simulink model "Nonlinear_model_with_observer"  (Simulink 7.7)
settings: Solver=ode45  StartTime=0.0  StopTime=6  RelTol=1e-3
undefined symbols (not defined in the file or in its folder): quad
settings Model: Creator=Alexey  LastModifiedBy=Alexey

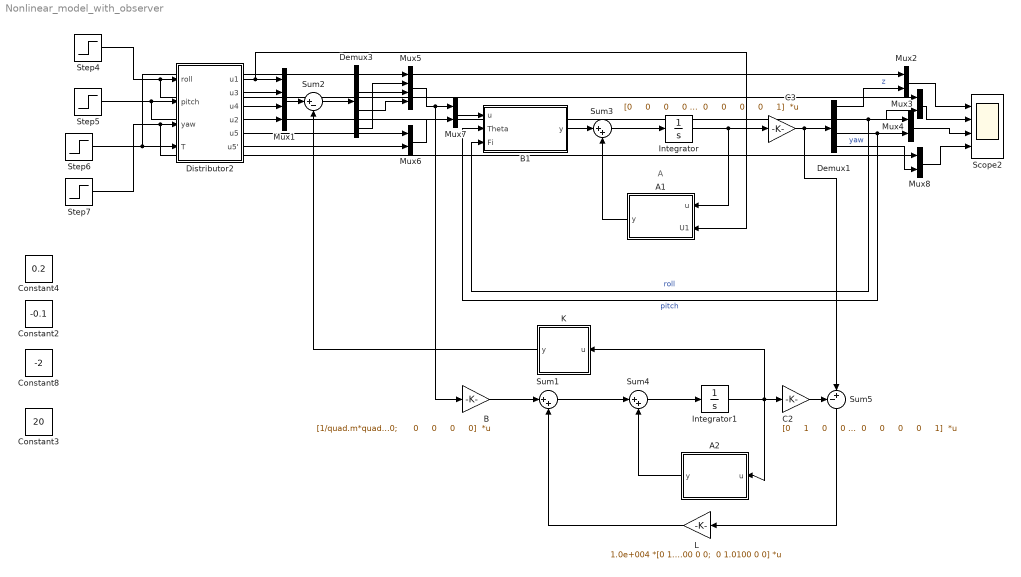
== system Nonlinear_model_with_observer ==
  note: A
  A1 : Stateflow chart  TreatAsAtomicUnit=on
  A2 : Stateflow chart  TreatAsAtomicUnit=on
  "B " : Gain  Gain=|  Multiplication=Matrix(K*u)
      | [1/quad.m*quad.b     0     0     0;
      |      0     0     0     0;
      |      0     0     1/quad.Ixx*quad.b*quad.l     0;
      |      0     0     0     0;
      |      0     0     0     1/quad.Iyy*quad.b*quad.l;
      |      0     0     0     0;
      |      0     1/quad.Izz*quad.k*quad.r     0     0;
      |      0     0     0     0]
  B1 : Stateflow chart  TreatAsAtomicUnit=on
  C2 : Gain  Gain=|  Multiplication=Matrix(K*u)
      | [0     1     0     0     0     0     0     0;
      |      0     0     0     1     0     0     0     0;
      |      0     0     0     0     0     1     0     0;
      |      0     0     0     0     0     0     0     1]
  C3 : Gain  Gain=|  Multiplication=Matrix(K*u)
      | [0     0     0     0     0     1     0     0     0     0     0     0;
      |      0     0     0     0     0     0     0     1     0     0     0     0;
      |      0     0     0     0     0     0     0     0     0     1     0     0;
      |      0     0     0     0     0     0     0     0     0     0     0     1]
  Constant2 : Constant  Value=-0.1
  Constant3 : Constant  Value=20
  Constant4 : Constant  Value=0.2
  Constant8 : Constant  Value=-2
  Demux1 : Demux
  Demux3 : Demux
  Distributor2 : Subsystem
  Integrator : Integrator  ZeroCross=off
  Integrator1 : Integrator
  K : Stateflow chart  TreatAsAtomicUnit=on
  L : Gain  Gain=|  Multiplication=Matrix(K*u)
      | 1.0e+004 *[0 1.0100 0 0; 
      | 0 1.0100 0 0; 
      | 0 1.0100 0 0; 
      | 0 1.0100 0 0; 
      | 0 1.0100 0 0; 
      | 0 1.0100 0 0; 
      | 0 1.0100 0 0; 
      | 0 1.0100 0 0]
  Mux1 : Mux
  Mux{2..4,6..8} (6 alike) : Mux  Inputs=2
  Mux5 : Mux
  Scope2 : Scope  NumInputPorts=4
      settings: TimeRange=1  YMin=9.95~0.0095~-0.0335~0.19  YMax=10.5~0.0135~-0.031~0.23
  Step4 : Step  Time=3.5  After=-0.1  SampleTime=0
  Step5 : Step  Time=3  Before=-0.2  After=0.1  SampleTime=0
  Step6 : Step  Time=2  After=2  SampleTime=0
  Step7 : Step  After=10  SampleTime=0
  Sum1 : Sum  Inputs=|++
  Sum2 : Sum  Inputs=|+-
  Sum3 : Sum  Inputs=|++
  Sum4 : Sum  Inputs=|++
  Sum5 : Sum  Inputs=-+|
  wires:
  B1/1(y) -> Sum3/1
  Sum3/1 -> Integrator/1
  Integrator/1 -> C3/1, A1/1(u)
  A1/1(y) -> Sum3/2
  Distributor2/1("u1 ") -> Mux1/1, A1/2(U1)
  Mux1/1 -> Sum2/1
  Sum2/1 -> Demux3/1
  Distributor2/5("u5 ") -> Mux6/1
  Distributor2/6(u5') -> Mux6/2
  Demux3/1 -> Mux5/1
  Demux3/4 -> Mux5/2
  Demux3/2 -> Mux5/3
  Distributor2/2("u3 ") -> Mux1/2
  Distributor2/3("u4 ") -> Mux1/3
  Distributor2/4("u2 ") -> Mux1/4
  Mux5/1 -> Mux7/1, "B "/1
  Mux6/1 -> Mux7/2
  Mux7/1 -> B1/1(u)
  Demux3/3 -> Mux5/4
  Demux1/1 -> Mux2/2  "z"
  Demux1/2 -> B1/3(Fi), Mux3/2  "roll"
  Demux1/3 -> B1/2(Theta), Mux4/2  "pitch"
  Demux1/4 -> Mux8/2  "yaw"
  C3/1 -> Demux1/1, Sum5/2
  Sum1/1 -> Sum4/1
  Sum4/1 -> Integrator1/1
  Integrator1/1 -> C2/1, K/1(u), A2/1(u)
  C2/1 -> Sum5/1
  A2/1(y) -> Sum4/2
  Sum5/1 -> L/1
  L/1 -> Sum1/2
  "B "/1 -> Sum1/1
  K/1(y) -> Sum2/2
  Step4/1 -> Distributor2/1(roll), Mux3/1
  Step5/1 -> Distributor2/2(pitch), Mux4/1
  Step6/1 -> Distributor2/3(yaw), Mux8/1
  Step7/1 -> Distributor2/4(T), Mux2/1
  Mux2/1 -> Scope2/1
  Mux8/1 -> Scope2/4
  Mux4/1 -> Scope2/3
  Mux3/1 -> Scope2/2

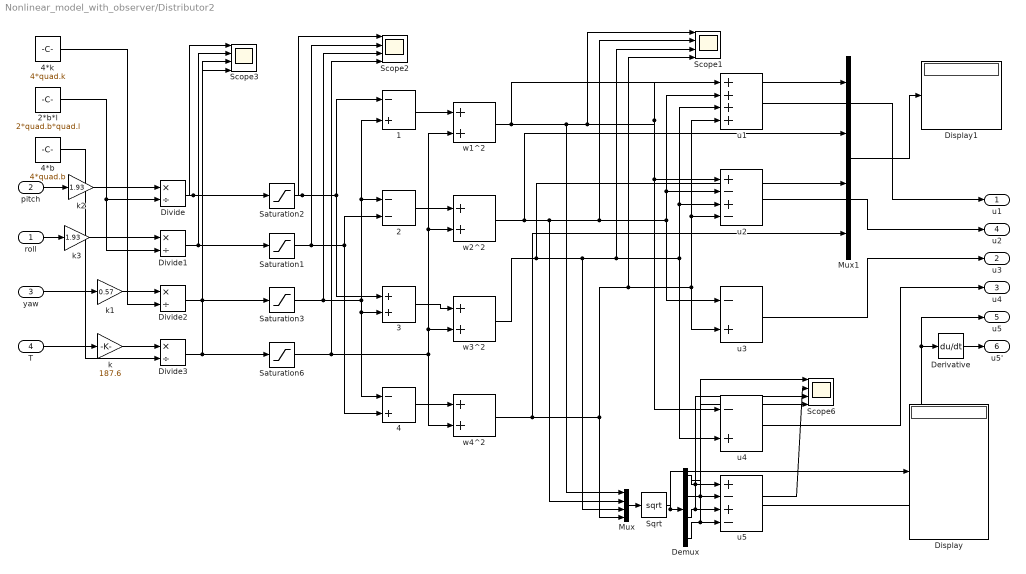
== system Nonlinear_model_with_observer/Distributor2 ==
  roll : Inport
  pitch : Inport  Port=2
  yaw : Inport  Port=3
  T : Inport  Port=4
  1 : Sum  Inputs=-+
  2 : Sum  Inputs=--
  2*b*l : Constant  Value=2*quad.b*quad.l
  3 : Sum
  4 : Sum  Inputs=-+
  4*b : Constant  Value=4*quad.b
  4*k : Constant  Value=4*quad.k
  Demux : Demux
  Derivative : Derivative
  Display : Display
  Display1 : Display
  Divide{,1..3} (4 alike) : Product  Inputs=*/
  Mux : Mux
  Mux1 : Mux
  Saturation1 : Saturate  UpperLimit=287850  LowerLimit=-287850
  Saturation2 : Saturate  UpperLimit=287850  LowerLimit=-287850
  Saturation3 : Saturate  UpperLimit=9000000000  LowerLimit=-9000000000  LinearizeAsGain=off
  Saturation6 : Saturate  UpperLimit=1574000000  LowerLimit=15740000
  Scope{1..3,6} (4 alike) : Scope  NumInputPorts=4
      Scope1 settings: TimeRange=1  YMin=-5~-5~-5~-5  YMax=5~5~5~5  SaveName=ScopeData2
      Scope2 settings: TimeRange=1  YMin=-5~-5~-5~-5  YMax=5~5~5~5  SaveName=ScopeData4
      Scope3 settings: TimeRange=1  YMin=-5~-5~-5~-5  YMax=5~5~5~5  SaveName=ScopeData5
      Scope6 settings: TimeRange=1  YMin=-5~-5~-5~-5  YMax=5~5~5~5  SaveName=ScopeData6
  Sqrt : Sqrt  SaturateOnIntegerOverflow=on
  k : Gain  Gain=187.6
  k1 : Gain  Gain=0.57
  k2 : Gain  Gain=1.93
  k3 : Gain  Gain=1.93
  u1 : Sum  Inputs=++++
  u2 : Sum  Inputs=+-+-
  u3 : Sum  Inputs=-+
  u4 : Sum  Inputs=-+
  u5 : Sum  Inputs=+-+-
  w1^2 : Sum
  w2^2 : Sum
  w3^2 : Sum
  w4^2 : Sum
  "u1 " : Outport
  "u3 " : Outport  Port=2
  "u4 " : Outport  Port=3
  "u2 " : Outport  Port=4
  "u5 " : Outport  Port=5
  u5' : Outport  Port=6
  wires:
  4*k/1 -> Divide2/2
  Divide1/1 -> Scope3/2, Saturation1/1
  Divide2/1 -> Scope3/3, Saturation3/1
  Divide/1 -> Scope3/1, Saturation2/1
  4*b/1 -> Divide3/2
  yaw/1 -> k1/1
  2*b*l/1 -> Divide/2, Divide1/2
  roll/1 -> k3/1
  pitch/1 -> k2/1
  w1^2/1 -> Mux/1, u1/1, u2/1, u4/1, Scope1/1, Mux1/1
  w2^2/1 -> Mux/2, u1/2, u2/2, u3/1, Scope1/2, Mux1/2
  w3^2/1 -> Mux/3, u1/3, u2/3, u4/2, Scope1/3, Mux1/3
  w4^2/1 -> Mux/4, u1/4, u2/4, u3/2, Scope1/4, Mux1/4
  Divide3/1 -> Scope3/4, Saturation6/1
  T/1 -> k/1
  u1/1 -> "u1 "/1
  u2/1 -> "u2 "/1
  u3/1 -> "u3 "/1
  u4/1 -> "u4 "/1
  Mux/1 -> Sqrt/1
  Sqrt/1 -> Demux/1, Display/1
  Demux/1 -> u5/1, Scope6/1
  Demux/3 -> u5/3, Scope6/3
  Demux/2 -> u5/2, Scope6/2
  Demux/4 -> u5/4, Scope6/4
  u5/1 -> Derivative/1, "u5 "/1
  Derivative/1 -> u5'/1
  1/1 -> w1^2/1
  2/1 -> w2^2/1
  3/1 -> w3^2/1
  4/1 -> w4^2/1
  Saturation6/1 -> w1^2/2, w2^2/2, w3^2/2, w4^2/2, Scope2/4
  Mux1/1 -> Display1/1
  Saturation2/1 -> 1/1, 3/1, Scope2/1
  Saturation1/1 -> 2/2, 4/2, Scope2/2
  Saturation3/1 -> 3/2, 4/1, 1/2, 2/1, Scope2/3
  k2/1 -> Divide/1
  k3/1 -> Divide1/1
  k1/1 -> Divide2/1
  k/1 -> Divide3/1

== matlab function K ==
  data: u input double; y output double
function y = fcn(u)
%#codegen

K=[9282000    62976000 0 0 0 0 0 0;
      0 0 889700     2896900 0 0 0 0;
      0 0 0 0 889700     2896900 0 0;
    0 0 0 0 0 0 33088000    30881000]*u;

y=sum(K,2);

== matlab function A2 ==
  data: u input double; y output double
function y = fcn(u)
%#codegen

m=0.468;
b=2.9800e-006;

A = [0     0     0     0     0     0     0     0;
     1     0     0     0     0     0     0     0;
     0     0     0     0     0     0     0     0;
     0     0     1     0     0     0     0     0;
     0     0     0     0     0     0     0     0;
     0     0     0     0     1     0     0     0;
     0     0     0     0     0     0     0     0;
     0     0     0     0     0     0     1     0]*u;
 
 y=sum(A,2);

== matlab function A1 ==
  data: u input double; y output double; U1 input double
function y = fcn(u,U1)
%#codegen

m=0.468;
b=2.9800e-006;

A = [0     0     0     0     0     0     0     0     0     1/m*b*U1     0     0;
     1     0     0     0     0     0     0     1/m*b*U1     0     0     0     0;
     0     0     0     0     0     0     0     0     0     0     0     0;
     0     0     1     0     0     0     0     0     0     0     0     0;
     0     0     0     0     0     0     0     0     0     0     0     0;
     0     0     0     0     1     0     0     0     0     0     0     0;
     0     0     0     0     0     0     0     0     0     0     0     0;
     0     0     0     0     0     0     1     0     0     0     0     0;
     0     0     0     0     0     0     0     0     0     0     0     0;
     0     0     0     0     0     0     0     0     1     0     0     0;
     0     0     0     0     0     0     0     0     0     0     0     0;
     0     0     0     0     0     0     0     0     0     0     1     0]*u;
 
 y=sum(A,2);

== matlab function B1 ==
  data: u input double; y output double; Theta input double; Fi input double
function y = fcn(u,Theta,Fi)
%#codegen

m=0.468;
b=2.9800e-006;
k= 1.1400e-007;
Jr= 3.2441e-005;
l=0.225;
Jxx=0.082;
Jyy=Jxx;
Jzz=0.149;

y = [1/m*b*Theta     0     0     0     0     0;
     0     0     0     0     0     0;
     1/m*b*Fi     0     0     0     0     0;
     0     0     0     0     0     0;
     1/m*b     0     0     0     0     0;
     0     0     0     0     0     0;
     0     0     1/Jxx*b*l     0     0     0;
     0     0     0     0     0     0;
     0     0     0     1/Jyy*b*l     0     0;
     0     0     0     0     0     0;
     0     1/Jzz*k     0     0     0     Jr;
     0     0     0     0     0     0]*u;
